simulink model "linmodel_eq1_discr_lqr_val"  (R2019a)
settings: Solver=VariableStepAuto  StartTime=0.0  StopTime=30  RelTol=1e-3
InitFcn:
  | lin_discr_model
undefined symbols (not defined in the file): A_eq1_d_val, B_eq1_d2_val, C_eq1_d_val, K1, L_val, Ts, xref
settings Model: Creator=jessi  LastModifiedBy=jessi

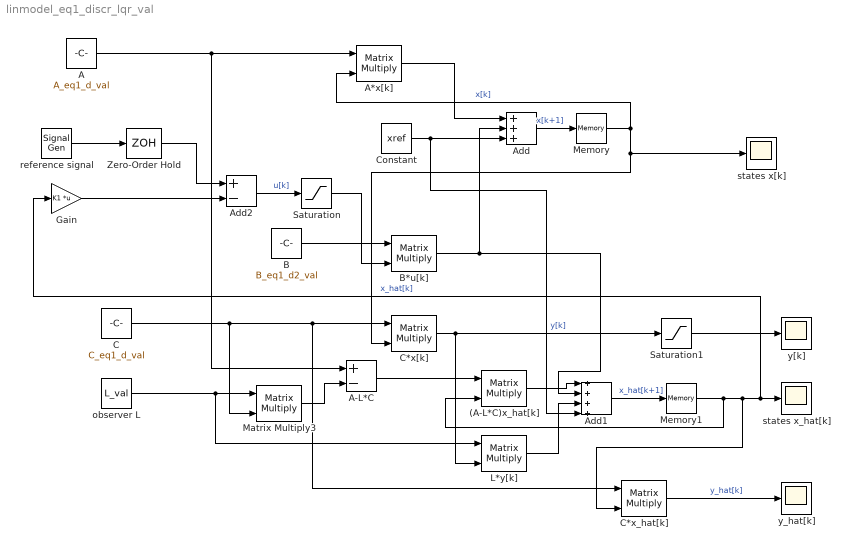
== system linmodel_eq1_discr_lqr_val ==
  (A-L*C)x_hat[k] : Product  Multiplication=Matrix(*)
  A : Constant  Value=A_eq1_d_val  SampleTime=Ts
  A*x[k] : Product  Multiplication=Matrix(*)
  A-L*C : Sum  Inputs=+-
  Add : Sum  Inputs=+++
  Add1 : Sum  Inputs=++++
  Add2 : Sum  Inputs=+-
  B : Constant  Value=B_eq1_d2_val  SampleTime=Ts
  B*u[k] : Product  Multiplication=Matrix(*)
  C : Constant  Value=C_eq1_d_val  SampleTime=Ts
  C*x[k] : Product  Multiplication=Matrix(*)
  C*x_hat[k] : Product  Multiplication=Matrix(*)
  Constant : Constant  Value=xref  SampleTime=Ts
  Gain : Gain  Gain=K1  Multiplication=Matrix(K*u)
  L*y[k] : Product  Multiplication=Matrix(*)
  Matrix Multiply3 : Product  Multiplication=Matrix(*)
  Memory : Memory  InitialCondition=[pi;0;0;0]
  Memory1 : Memory  InitialCondition=[pi;0;0;0]
  Saturation : Saturate  UpperLimit=10  LowerLimit=-10
  Saturation1 : Saturate  UpperLimit=2*pi  LowerLimit=-2*pi
  Zero-Order Hold : ZeroOrderHold  SampleTime=Ts
  observer L : Constant  Value=L_val  SampleTime=Ts
  reference signal : SignalGenerator  WaveForm=square  Amplitude=-0.3
  states x[k] : Scope
  states x_hat[k] : Scope
  y[k] : Scope
  y_hat[k] : Scope
  wires:
  B/1 -> B*u[k]/1
  A/1 -> A*x[k]/1, A-L*C/1
  A*x[k]/1 -> Add/1
  B*u[k]/1 -> Add1/2, Add/2
  Memory/1 -> A*x[k]/2, states x[k]/1, C*x[k]/2  "x[k]"
  C/1 -> Matrix Multiply3/2, C*x_hat[k]/1, C*x[k]/1
  C*x[k]/1 -> L*y[k]/2, Saturation1/1  "y[k]"
  observer L/1 -> L*y[k]/1, Matrix Multiply3/1
  Matrix Multiply3/1 -> A-L*C/2
  A-L*C/1 -> (A-L*C)x_hat[k]/1
  (A-L*C)x_hat[k]/1 -> Add1/1
  L*y[k]/1 -> Add1/3
  Add1/1 -> Memory1/1  "x_hat[k+1]"
  Memory1/1 -> (A-L*C)x_hat[k]/2, C*x_hat[k]/2, Gain/1, states x_hat[k]/1  "x_hat[k]"
  C*x_hat[k]/1 -> y_hat[k]/1  "y_hat[k]"
  Add/1 -> Memory/1  "x[k+1]"
  Constant/1 -> Add1/4, Add/3
  Add2/1 -> Saturation/1  "u[k]"
  Saturation/1 -> B*u[k]/2
  Saturation1/1 -> y[k]/1
  Zero-Order Hold/1 -> Add2/1
  reference signal/1 -> Zero-Order Hold/1
  Gain/1 -> Add2/2
